simulink model "DFA_PID_Controller_ESC"  (R2014a)
settings: Solver=ode4  StartTime=0.0  StopTime=Tfinal  FixedStep=Tstep  MaxStep=Tstep  RelTol=1e-7
values from neighbouring files (symbols this model uses):
  Accelmean = 0    [Script_DFA_PID_Controller_ESC.m]
  alpha0 = 0    [Script_DFA_PID_Controller_ESC.m]
  alpha_desired = 0.1    [Script_DFA_PID_Controller_ESC.m]
  beta0 = 0    [Script_DFA_PID_Controller_ESC.m]
  ci = [-.01235; -.01235; .01235; .01235]    [Script_DFA_PID_Controller_ESC.m]
  f0 = mg    [Script_DFA_PID_Controller_ESC.m]
  g = 9.806    [Script_DFA_PID_Controller_ESC.m]
  gamma0 = 0    [Script_DFA_PID_Controller_ESC.m]
  Gyromean = 0    [Script_DFA_PID_Controller_ESC.m]
  IR_mean = 0    [Script_DFA_PID_Controller_ESC.m]
  Ix = .004738    (= 0.004738)    [Script_DFA_PID_Controller_ESC.m]
  Ixy = Ix-Iy    (= -0.006032)    [Script_DFA_PID_Controller_ESC.m]
  Iy = .01077    (= 0.01077)    [Script_DFA_PID_Controller_ESC.m]
  Iyz = Iy-Iz    (= -0.0041)    [Script_DFA_PID_Controller_ESC.m]
  Iz = .01487    (= 0.01487)    [Script_DFA_PID_Controller_ESC.m]
  Izx = Iz-Ix    (= 0.010132)    [Script_DFA_PID_Controller_ESC.m]
  Kd_alpha = 60    [Script_DFA_PID_Controller_ESC.m]
  Kd_beta = 30    [Script_DFA_PID_Controller_ESC.m]
  Kd_gamma = 30    [Script_DFA_PID_Controller_ESC.m]
  Kd_x = 0.008    [Script_DFA_PID_Controller_ESC.m]
  Kd_y = 0.002    [Script_DFA_PID_Controller_ESC.m]
  Kd_z = 100    [Script_DFA_PID_Controller_ESC.m]
  Ki_alpha = 0    [Script_DFA_PID_Controller_ESC.m]
  Ki_beta = 0    [Script_DFA_PID_Controller_ESC.m]
  Ki_gamma = 0    [Script_DFA_PID_Controller_ESC.m]
  Ki_x = 0    [Script_DFA_PID_Controller_ESC.m]
  Ki_y = 0    [Script_DFA_PID_Controller_ESC.m]
  Ki_z = 200    [Script_DFA_PID_Controller_ESC.m]
  Kp_alpha = 50    [Script_DFA_PID_Controller_ESC.m]
  Kp_beta = 8    [Script_DFA_PID_Controller_ESC.m]
  Kp_gamma = 15    [Script_DFA_PID_Controller_ESC.m]
  Kp_x = .1    (= 0.1)    [Script_DFA_PID_Controller_ESC.m]
  Kp_y = .15    (= 0.15)    [Script_DFA_PID_Controller_ESC.m]
  Kp_z = 200    [Script_DFA_PID_Controller_ESC.m]
  m_total = sum(m)    [Script_DFA_PID_Controller_ESC.m]
  p0 = omega(1)    [Script_DFA_PID_Controller_ESC.m]
  poly_order = 1    [Script_DFA_PID_Controller_ESC.m]
  q0 = omega(2)    [Script_DFA_PID_Controller_ESC.m]
  r0 = omega(3)    [Script_DFA_PID_Controller_ESC.m]
  salpha = (2*10^-4)*(pi/180)    (= 3.49065850399e-06)    [Script_DFA_PID_Controller_ESC.m]
  salphadot = (5.7*10^-4)*(pi/180)    (= 9.94837673637e-06)    [Script_DFA_PID_Controller_ESC.m]
  sbeta = (2*10^-4)*(pi/180)    (= 3.49065850399e-06)    [Script_DFA_PID_Controller_ESC.m]
  sbetadot = (5.4*10^-4)*(pi/180)    (= 9.42477796077e-06)    [Script_DFA_PID_Controller_ESC.m]
  SENS_NOISE01 = 1    [Script_DFA_PID_Controller_ESC.m]
  sgamma = (2*10^-4)*(pi/180)    (= 3.49065850399e-06)    [Script_DFA_PID_Controller_ESC.m]
  sgammadot = (5.4*10^-4)*(pi/180)    (= 9.42477796077e-06)    [Script_DFA_PID_Controller_ESC.m]
  sx = (3*10^-4)/1000    (= 3e-07)    [Script_DFA_PID_Controller_ESC.m]
  sxdot = (3*10^-2)*(pi/180)    (= 0.000523598775598)    [Script_DFA_PID_Controller_ESC.m]
  sy = (3*10^-4)/1000    (= 3e-07)    [Script_DFA_PID_Controller_ESC.m]
  sydot = (3*10^-2)*(pi/180)    (= 0.000523598775598)    [Script_DFA_PID_Controller_ESC.m]
  sz = (5.8*10^-3)/1000    (= 5.8e-06)    [Script_DFA_PID_Controller_ESC.m]
  ThreeD_mean = 0    [Script_DFA_PID_Controller_ESC.m]
  vect_xi = [ -.154;     .154;      0;      0]    [Script_DFA_PID_Controller_ESC.m]
  vect_yi = [     0;        0;   .087;  -.087]    [Script_DFA_PID_Controller_ESC.m]
  x0 = 0    [Script_DFA_PID_Controller_ESC.m]
  x0dot = 0    [Script_DFA_PID_Controller_ESC.m]
  y0 = 0    [Script_DFA_PID_Controller_ESC.m]
  y0dot = 0    [Script_DFA_PID_Controller_ESC.m]
  z0 = 0    [Script_DFA_PID_Controller_ESC.m]
  z0dot = 0    [Script_DFA_PID_Controller_ESC.m]
  z_desired = 0.25    [Script_DFA_PID_Controller_ESC.m]
settings Model: Creator=colempT430  LastModifiedBy=Young
settings DataIOCC: SignalLoggingSaveFormat=ModelDataLogs
settings OptimizationCC: ExpressionDepthLimit=2147483647
settings DebuggingCC: UnderspecifiedInitializationDetection=Classic  FcnCallInpInsideContextMsg=EnableAllAsWarning  StateNameClashWarn=warning

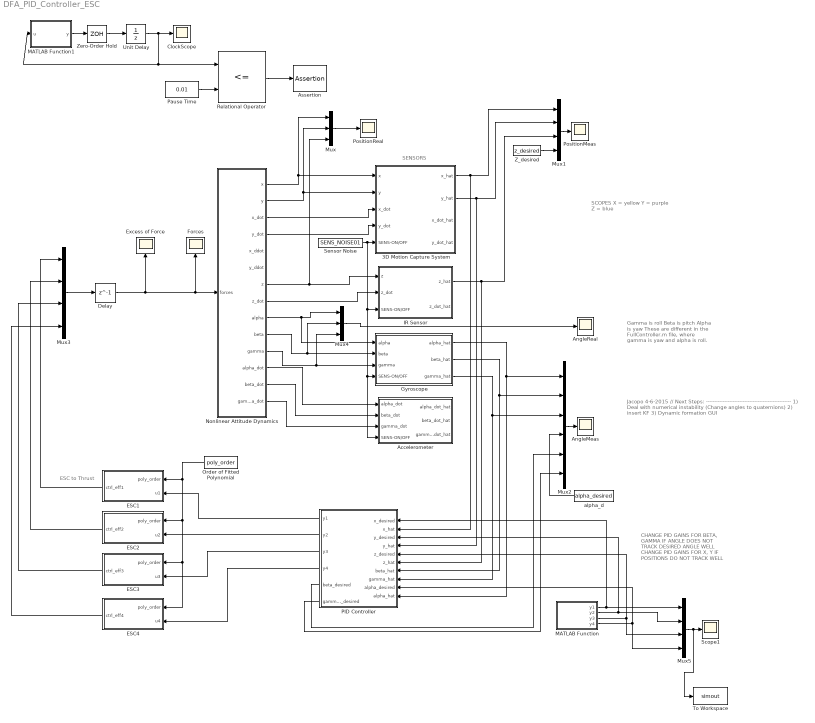
== system DFA_PID_Controller_ESC ==
  note: CHANGE PID GAINS FOR
      | BETA, GAMMA IF ANGLE
      | DOES NOT TRACK DESIRED
      | ANGLE WELL
      |
      | CHANGE PID GAINS FOR
      | X, Y IF POSITIONS DO NOT
      | TRACK WELL
  note: ESC to Thrust
  note: SENSORS
  note: SCOPES
      |
      | X = yellow
      | Y = purple
      | Z = blue
  note: Gamma is roll
      | Beta is pitch
      | Alpha is yaw
      |
      | These are different in the FullController.m file, where gamma is yaw and alpha is roll.
  note: Jacopo 4-6-2015 // Next Steps:
      | ---------------------------------------------------
      | 1) Deal with numerical instability (Change angles to quaternions)
      | 2) insert KF
      | 3) Dynamic formation GUI
  3D Motion Capture System : Subsystem
  Accelerometer : Subsystem
  AngleMeas : Scope
      settings: YMin=-0.25  YMax=0.4  SaveName=PositionMeas1
  AngleReal : Scope
      settings: YMin=-0.25  YMax=0.4  SaveName=PositionMeas2
  Assertion : Assertion  AssertionFailFcn=set_param(bdroot, 'SimulationCommand', 'pause')  StopWhenAssertionFail=off
  ClockScope : Scope
      settings: SaveName=NclockData
  Delay : Delay  DelayLength=1  InitialCondition=f0
  ESC1 : MATLAB Function  TreatAsAtomicUnit=on
  ESC2 : MATLAB Function  TreatAsAtomicUnit=on
  ESC3 : MATLAB Function  TreatAsAtomicUnit=on
  ESC4 : MATLAB Function  TreatAsAtomicUnit=on
  Excess of Force : Scope
      settings: SaveName=input_u
  Forces : Scope
      settings: SaveName=input_u1
  Gyroscope : Subsystem
  IR Sensor : Subsystem
  MATLAB Function : MATLAB Function  TreatAsAtomicUnit=on
  MATLAB Function1 : MATLAB Function  TreatAsAtomicUnit=on
  Mux : Mux  Inputs=3
  Mux1 : Mux
  Mux2 : Mux  Inputs=6
  Mux3 : Mux
  Mux4 : Mux  Inputs=3
  Mux5 : Mux
  Nonlinear Attitude Dynamics : Subsystem
  Order of Fitted Polynomial : Constant  Value=poly_order
  PID Controller : Subsystem
  Pause Time : Constant  Value=0.01
  PositionMeas : Scope
      settings: YMin=-0.025  YMax=0.5  SaveName=PositionMeas
  PositionReal : Scope
      settings: YMin=0  YMax=0.275  SaveName=PositionReal
  Relational Operator : RelationalOperator  Operator=<=  OutDataTypeStr=boolean
  Scope1 : Scope
  Sensor Noise : Constant  Value=SENS_NOISE01
  To Workspace : ToWorkspace  VariableName=simout  SampleTime=-1
      settings: Save2DSignal=2-D array (concatenate along first dimension)
  Unit Delay : UnitDelay  SampleTime=-1
  Z_desired : Constant  Value=z_desired
  Zero-Order Hold : ZeroOrderHold  SampleTime=-1
  alpha_d : Constant  Value=alpha_desired
  wires:
  Nonlinear Attitude Dynamics/1(x) -> 3D Motion Capture System/1(x), Mux/1
  Nonlinear Attitude Dynamics/2(y) -> 3D Motion Capture System/2(y), Mux/2
  Nonlinear Attitude Dynamics/7(z) -> IR Sensor/1(z), Mux/3
  Nonlinear Attitude Dynamics/9(alpha) -> Gyroscope/1(alpha), Mux4/1
  Nonlinear Attitude Dynamics/10(beta) -> Gyroscope/2(beta), Mux4/2
  Nonlinear Attitude Dynamics/11(gamma) -> Gyroscope/3(gamma), Mux4/3
  Nonlinear Attitude Dynamics/13(beta_dot) -> Accelerometer/2(beta_dot)
  3D Motion Capture System/1(x_hat) -> PID Controller/2(x_hat), Mux1/1
  IR Sensor/1(z_hat) -> PID Controller/6(z_hat), Mux1/3
  3D Motion Capture System/2(y_hat) -> PID Controller/4(y_hat), Mux1/2
  Gyroscope/2(beta_hat) -> PID Controller/7(beta_hat), Mux2/2
  Nonlinear Attitude Dynamics/3(x_dot) -> 3D Motion Capture System/3(x_dot)
  Nonlinear Attitude Dynamics/4(y_dot) -> 3D Motion Capture System/4(y_dot)
  Nonlinear Attitude Dynamics/8(z_dot) -> IR Sensor/2(z_dot)
  Mux/1 -> PositionReal/1
  Mux1/1 -> PositionMeas/1
  Sensor Noise/1 -> 3D Motion Capture System/5(SENS-ON/OFF), Accelerometer/4(SENS-ON/OFF), Gyroscope/4(SENS-ON/OFF), IR Sensor/3(SENS-ON/OFF)
  Gyroscope/1(alpha_hat) -> PID Controller/10(alpha_hat), Mux2/1
  Gyroscope/3(gamma_hat) -> Mux2/3, PID Controller/8(gamma_hat)
  MATLAB Function/4(y4) -> Mux5/4, PID Controller/9(alpha_desired)
  Mux2/1 -> AngleMeas/1
  Z_desired/1 -> Mux1/4
  alpha_d/1 -> Mux2/4
  PID Controller/5(beta_desired) -> Mux2/5
  PID Controller/6(gamma_desired) -> Mux2/6
  Nonlinear Attitude Dynamics/12(alpha_dot) -> Accelerometer/1(alpha_dot)
  Nonlinear Attitude Dynamics/14(gamma_dot) -> Accelerometer/3(gamma_dot)
  MATLAB Function/1(y1) -> Mux5/1, PID Controller/1(x_desired)
  Order of Fitted Polynomial/1 -> ESC4/1(poly_order), ESC3/1(poly_order), ESC2/1(poly_order), ESC1/1(poly_order)
  Delay/1 -> Forces/1, Nonlinear Attitude Dynamics/1(forces), Excess of Force/1
  Mux3/1 -> Delay/1
  ESC2/1(ctrl_eff2) -> Mux3/2
  ESC3/1(ctrl_eff3) -> Mux3/3
  ESC4/1(ctrl_eff4) -> Mux3/4
  ESC1/1(ctrl_eff1) -> Mux3/1
  PID Controller/1(y1) -> ESC1/2(u1)
  PID Controller/2(y2) -> ESC2/2(u2)
  PID Controller/3(y3) -> ESC3/2(u3)
  PID Controller/4(y4) -> ESC4/2(u4)
  Mux4/1 -> AngleReal/1
  MATLAB Function/2(y2) -> Mux5/2, PID Controller/3(y_desired)
  MATLAB Function/3(y3) -> Mux5/3, PID Controller/5(z_desired)
  Pause Time/1 -> Relational Operator/2
  Relational Operator/1 -> Assertion/1
  Zero-Order Hold/1 -> Unit Delay/1
  MATLAB Function1/1(y) -> Zero-Order Hold/1
  Unit Delay/1 -> Relational Operator/1, MATLAB Function1/1(u), ClockScope/1
  Mux5/1 -> To Workspace/1, Scope1/1

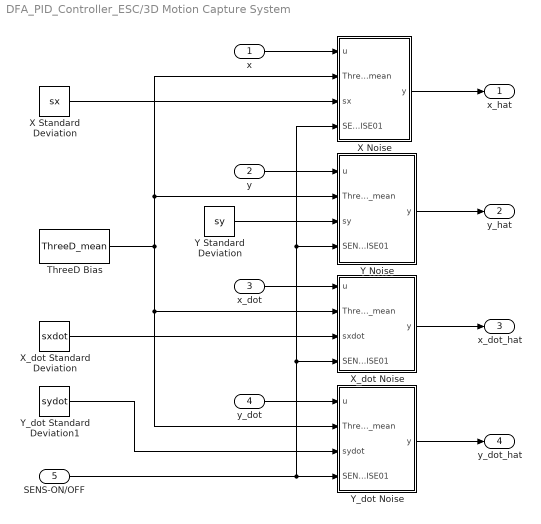
== system DFA_PID_Controller_ESC/3D Motion Capture System ==
  x : Inport
  y : Inport  Port=2
  x_dot : Inport  Port=3
  y_dot : Inport  Port=4
  SENS-ON/OFF : Inport  Port=5
  ThreeD Bias : Constant  Value=ThreeD_mean
  X Noise : MATLAB Function  TreatAsAtomicUnit=on
  X Standard Deviation : Constant  Value=sx
  X_dot Noise : MATLAB Function  TreatAsAtomicUnit=on
  X_dot Standard Deviation : Constant  Value=sxdot
  Y Noise : MATLAB Function  TreatAsAtomicUnit=on
  Y Standard Deviation : Constant  Value=sy
  Y_dot Noise : MATLAB Function  TreatAsAtomicUnit=on
  Y_dot Standard Deviation1 : Constant  Value=sydot
  x_hat : Outport
  y_hat : Outport  Port=2
  x_dot_hat : Outport  Port=3
  y_dot_hat : Outport  Port=4
  wires:
  x/1 -> X Noise/1(u)
  X Noise/1(y) -> x_hat/1
  y/1 -> Y Noise/1(u)
  Y Noise/1(y) -> y_hat/1
  x_dot/1 -> X_dot Noise/1(u)
  X_dot Noise/1(y) -> x_dot_hat/1
  y_dot/1 -> Y_dot Noise/1(u)
  Y_dot Noise/1(y) -> y_dot_hat/1
  X Standard Deviation/1 -> X Noise/3(sx)
  X_dot Standard Deviation/1 -> X_dot Noise/3(sxdot)
  ThreeD Bias/1 -> X Noise/2(ThreeD_mean), Y Noise/2(ThreeD_mean), Y_dot Noise/2(ThreeD_mean), X_dot Noise/2(ThreeD_mean)
  SENS-ON/OFF/1 -> X Noise/4(SENS_NOISE01), Y Noise/4(SENS_NOISE01), X_dot Noise/4(SENS_NOISE01), Y_dot Noise/4(SENS_NOISE01)
  Y Standard Deviation/1 -> Y Noise/3(sy)
  Y_dot Standard Deviation1/1 -> Y_dot Noise/3(sydot)

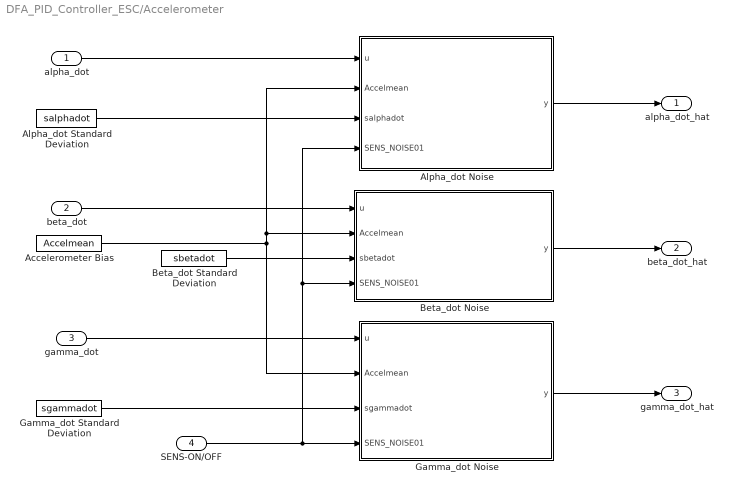
== system DFA_PID_Controller_ESC/Accelerometer ==
  alpha_dot : Inport
  beta_dot : Inport  Port=2
  gamma_dot : Inport  Port=3
  SENS-ON/OFF : Inport  Port=4
  Accelerometer Bias : Constant  Value=Accelmean
  Alpha_dot Noise : MATLAB Function  TreatAsAtomicUnit=on
  Alpha_dot Standard Deviation : Constant  Value=salphadot
  Beta_dot Noise : MATLAB Function  TreatAsAtomicUnit=on
  Beta_dot Standard Deviation : Constant  Value=sbetadot
  Gamma_dot Noise : MATLAB Function  TreatAsAtomicUnit=on
  Gamma_dot Standard Deviation : Constant  Value=sgammadot
  alpha_dot_hat : Outport
  beta_dot_hat : Outport  Port=2
  gamma_dot_hat : Outport  Port=3
  wires:
  beta_dot/1 -> Beta_dot Noise/1(u)
  gamma_dot/1 -> Gamma_dot Noise/1(u)
  Beta_dot Noise/1(y) -> beta_dot_hat/1
  Gamma_dot Noise/1(y) -> gamma_dot_hat/1
  alpha_dot/1 -> Alpha_dot Noise/1(u)
  Alpha_dot Noise/1(y) -> alpha_dot_hat/1
  Accelerometer Bias/1 -> Alpha_dot Noise/2(Accelmean), Beta_dot Noise/2(Accelmean), Gamma_dot Noise/2(Accelmean)
  Gamma_dot Standard Deviation/1 -> Gamma_dot Noise/3(sgammadot)
  Alpha_dot Standard Deviation/1 -> Alpha_dot Noise/3(salphadot)
  Beta_dot Standard Deviation/1 -> Beta_dot Noise/3(sbetadot)
  SENS-ON/OFF/1 -> Gamma_dot Noise/4(SENS_NOISE01), Beta_dot Noise/4(SENS_NOISE01), Alpha_dot Noise/4(SENS_NOISE01)

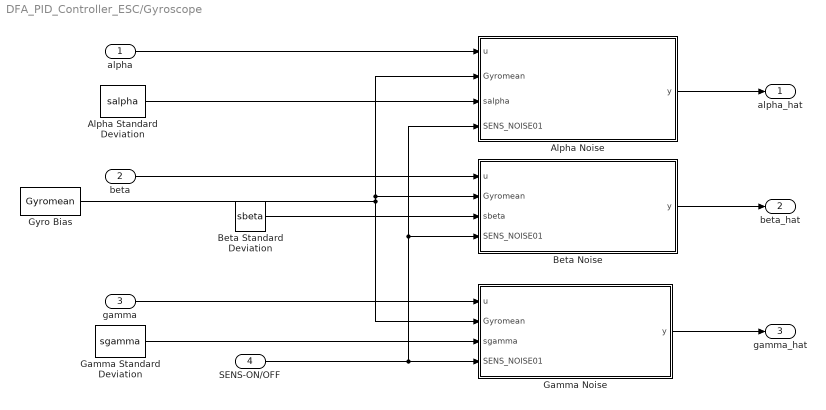
== system DFA_PID_Controller_ESC/Gyroscope ==
  alpha : Inport
  beta : Inport  Port=2
  gamma : Inport  Port=3
  SENS-ON/OFF : Inport  Port=4
  Alpha Noise : MATLAB Function  TreatAsAtomicUnit=on
  Alpha Standard Deviation : Constant  Value=salpha
  Beta Noise : MATLAB Function  TreatAsAtomicUnit=on
  Beta Standard Deviation : Constant  Value=sbeta
  Gamma Noise : MATLAB Function  TreatAsAtomicUnit=on
  Gamma Standard Deviation : Constant  Value=sgamma
  Gyro Bias : Constant  Value=Gyromean
  alpha_hat : Outport
  beta_hat : Outport  Port=2
  gamma_hat : Outport  Port=3
  wires:
  gamma/1 -> Gamma Noise/1(u)
  Gamma Noise/1(y) -> gamma_hat/1
  Alpha Noise/1(y) -> alpha_hat/1
  Beta Noise/1(y) -> beta_hat/1
  beta/1 -> Beta Noise/1(u)
  alpha/1 -> Alpha Noise/1(u)
  Alpha Standard Deviation/1 -> Alpha Noise/3(salpha)
  Beta Standard Deviation/1 -> Beta Noise/3(sbeta)
  Gamma Standard Deviation/1 -> Gamma Noise/3(sgamma)
  Gyro Bias/1 -> Alpha Noise/2(Gyromean), Beta Noise/2(Gyromean), Gamma Noise/2(Gyromean)
  SENS-ON/OFF/1 -> Beta Noise/4(SENS_NOISE01), Alpha Noise/4(SENS_NOISE01), Gamma Noise/4(SENS_NOISE01)

== system DFA_PID_Controller_ESC/IR Sensor ==
  z : Inport
  z_dot : Inport  Port=2
  SENS-ON/OFF : Inport  Port=3
  IR Bias : Constant  Value=IR_mean
  Z Noise : MATLAB Function  TreatAsAtomicUnit=on
  Z Standard Deviation : Constant  Value=sz
  Z_dot Noise : MATLAB Function  TreatAsAtomicUnit=on
  z_hat : Outport
  z_dot_hat : Outport  Port=2
  wires:
  z/1 -> Z Noise/1(u)
  Z Noise/1(y) -> z_hat/1
  z_dot/1 -> Z_dot Noise/1(u)
  Z_dot Noise/1(y) -> z_dot_hat/1
  Z Standard Deviation/1 -> Z_dot Noise/3(sz), Z Noise/3(sz)
  IR Bias/1 -> Z_dot Noise/2(IR_mean), Z Noise/2(IR_mean)
  SENS-ON/OFF/1 -> Z_dot Noise/4(SENS_NOISE01), Z Noise/4(SENS_NOISE01)

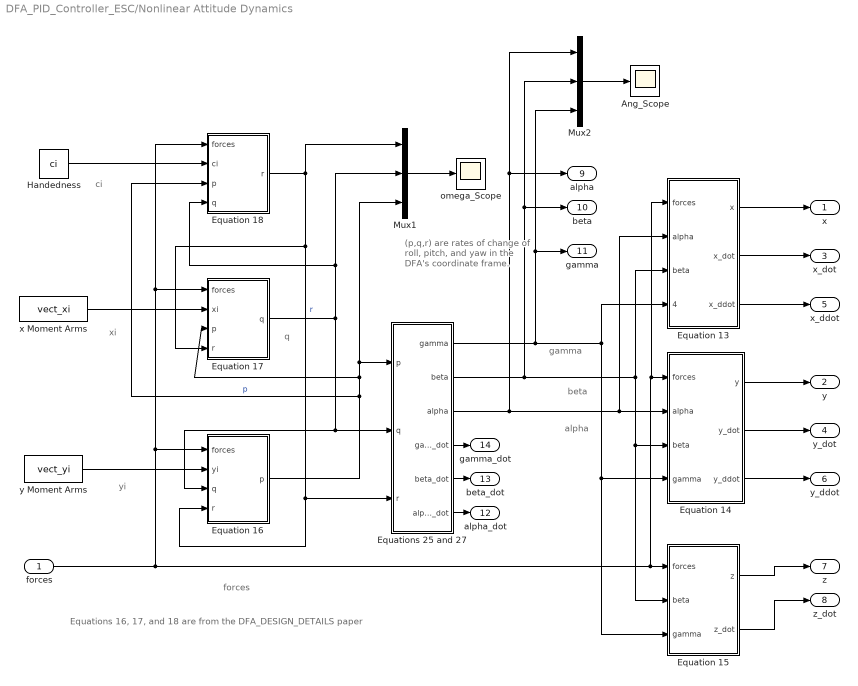
== system DFA_PID_Controller_ESC/Nonlinear Attitude Dynamics ==
  note: gamma
  note: Equations 16, 17, and 18 are from the DFA_DESIGN_DETAILS paper
  note: (p,q,r) are rates of change of roll, pitch, and yaw in the DFA's coordinate frame.
  note: forces
  note: yi
  note: xi
  note: ci
  note: q
  note: beta
  note: alpha
  forces : Inport
  Ang_Scope : Scope
      settings: SaveName=Ang_Scope1
  Equation 13 : Subsystem
  Equation 14 : Subsystem
  Equation 15 : Subsystem
  Equation 16 : Subsystem
  Equation 17 : Subsystem
  Equation 18 : Subsystem
  Equations 25 and 27 : Subsystem
  Handedness : Constant  Value=ci
  Mux1 : Mux  Inputs=3
  Mux2 : Mux  Inputs=3
  omega_Scope : Scope
      settings: SaveName=angle_Scope1
  x Moment Arms : Constant  Value=vect_xi
  y Moment Arms : Constant  Value=vect_yi
  x : Outport
  y : Outport  Port=2
  x_dot : Outport  Port=3
  y_dot : Outport  Port=4
  x_ddot : Outport  Port=5
  y_ddot : Outport  Port=6
  z : Outport  Port=7
  z_dot : Outport  Port=8
  alpha : Outport  Port=9
  beta : Outport  Port=10
  gamma : Outport  Port=11
  alpha_dot : Outport  Port=12
  beta_dot : Outport  Port=13
  gamma_dot : Outport  Port=14
  wires:
  Equation 18/1(r) -> Equations 25 and 27/3(r), Equation 16/4(r), Equation 17/4(r), Mux1/1  "r"
  Equation 16/1(p) -> Equation 18/3(p), Equations 25 and 27/1(p), Mux1/3, Equation 17/3(p)  "p"
  Handedness/1 -> Equation 18/2(ci)
  Equation 13/1(x) -> x/1
  Equation 14/1(y) -> y/1
  Equation 15/1(z) -> z/1
  Mux1/1 -> omega_Scope/1
  x Moment Arms/1 -> Equation 17/2(xi)
  Equation 17/1(q) -> Equations 25 and 27/2(q), Equation 16/3(q), Equation 18/4(q), Mux1/2
  y Moment Arms/1 -> Equation 16/2(yi)
  Equations 25 and 27/1(gamma) -> Equation 15/3(gamma), Equation 14/4(gamma), Equation 13/4(gamma), Mux2/3, gamma/1
  Equations 25 and 27/2(beta) -> Equation 15/2(beta), Equation 14/3(beta), Equation 13/3(beta), Mux2/2, beta/1
  Equations 25 and 27/3(alpha) -> Equation 13/2(alpha), Equation 14/2(alpha), Mux2/1, alpha/1
  Equations 25 and 27/4(gamma_dot) -> gamma_dot/1
  Equations 25 and 27/5(beta_dot) -> beta_dot/1
  Equations 25 and 27/6(alpha_dot) -> alpha_dot/1
  Equation 13/2(x_dot) -> x_dot/1
  Equation 14/2(y_dot) -> y_dot/1
  Equation 15/2(z_dot) -> z_dot/1
  forces/1 -> Equation 18/1(forces), Equation 17/1(forces), Equation 16/1(forces), Equation 13/1(forces), Equation 14/1(forces), Equation 15/1(forces)
  Mux2/1 -> Ang_Scope/1
  Equation 13/3(x_ddot) -> x_ddot/1
  Equation 14/3(y_ddot) -> y_ddot/1

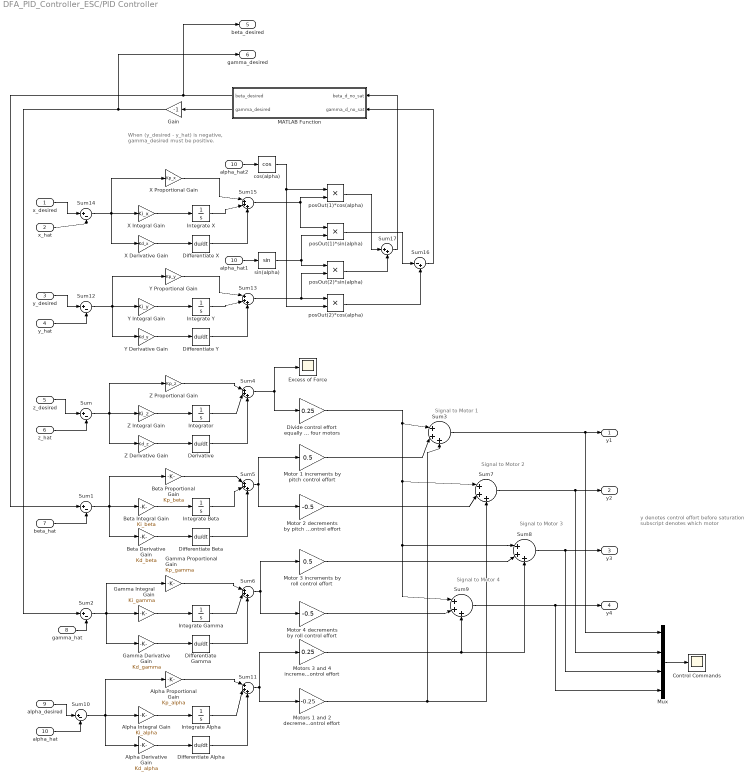
== system DFA_PID_Controller_ESC/PID Controller ==
  note: When (y_desired - y_hat) is negative,
      | gamma_desired must be positive.
  note: y denotes control effort before saturation
      | subscript denotes which motor
  note: Signal to Motor 4
  note: Signal to Motor 3
  note: Signal to Motor 2
  note: Signal to Motor 1
  x_desired : Inport
  x_hat : Inport  Port=2
  y_desired : Inport  Port=3
  y_hat : Inport  Port=4
  z_desired : Inport  Port=5
  z_hat : Inport  Port=6
  beta_hat : Inport  Port=7
  gamma_hat : Inport  Port=8
  alpha_desired : Inport  Port=9
  alpha_hat : Inport  Port=10
  Alpha Derivative Gain : Gain  Gain=Kd_alpha
  Alpha Integral Gain : Gain  Gain=Ki_alpha
  Alpha Proportional Gain : Gain  Gain=Kp_alpha
  Beta Derivative Gain : Gain  Gain=Kd_beta
  Beta Integral Gain : Gain  Gain=Ki_beta
  Beta Proportional Gain : Gain  Gain=Kp_beta
  Control Commands : Scope
      settings: SaveName=ControlCommandScope
  Derivative : Derivative
  Differentiate Alpha : Derivative
  Differentiate Beta : Derivative
  Differentiate Gamma : Derivative
  Differentiate X : Derivative
  Differentiate Y : Derivative
  Divide control effort equally among the four motors : Gain  Gain=0.25
  Excess of Force : Scope
      settings: SaveName=ExcessForce
  Gain : Gain  Gain=-1
  Gamma Derivative Gain : Gain  Gain=Kd_gamma
  Gamma Integral Gain : Gain  Gain=Ki_gamma
  Gamma Proportional Gain : Gain  Gain=Kp_gamma
  Integrate Alpha : Integrator
  Integrate Beta : Integrator
  Integrate Gamma : Integrator
  Integrate X : Integrator
  Integrate Y : Integrator
  Integrator : Integrator
  MATLAB Function : MATLAB Function  TreatAsAtomicUnit=on
  Motor 1 increments by pitch control effort : Gain  Gain=0.5
  Motor 2 decrements by pitch control effort : Gain  Gain=-0.5
  Motor 3 increments by roll control effort : Gain  Gain=0.5
  Motor 4 decrements by roll control effort : Gain  Gain=-0.5
  Motors 1 and 2 decrement by the pitch control effort : Gain  Gain=-0.25
  Motors 3 and 4 increment by the pitch control effort : Gain  Gain=0.25
  Mux : Mux
  Sum{,1..2,10,12,14} (6 alike) : Sum  Inputs=|+-
  Sum{3..9,11,13,15} (10 alike) : Sum  Inputs=|+++
  Sum16 : Sum  Inputs=|-+
  Sum17 : Sum  Inputs=|++
  X Derivative Gain : Gain  Gain=Kd_x
  X Integral Gain : Gain  Gain=Ki_x
  X Proportional Gain : Gain  Gain=Kp_x
  Y Derivative Gain : Gain  Gain=Kd_y
  Y Integral Gain : Gain  Gain=Ki_y
  Y Proportional Gain : Gain  Gain=Kp_y
  Z Derivative Gain : Gain  Gain=Kd_z
  Z Integral Gain : Gain  Gain=Ki_z
  Z Proportional Gain : Gain  Gain=Kp_z
  alpha_hat1 : InportShadow  Port=10
  alpha_hat2 : InportShadow  Port=10
  cos(alpha) : Trigonometry  Operator=cos
  posOut(1)*cos(alpha) : Product
  posOut(1)*sin(alpha) : Product
  posOut(2)*cos(alpha) : Product
  posOut(2)*sin(alpha) : Product
  sin(alpha) : Trigonometry
  y1 : Outport
  y2 : Outport  Port=2
  y3 : Outport  Port=3
  y4 : Outport  Port=4
  beta_desired : Outport  Port=5
  gamma_desired : Outport  Port=6
  wires:
  z_desired/1 -> Sum/1
  z_hat/1 -> Sum/2
  beta_hat/1 -> Sum1/2
  gamma_hat/1 -> Sum2/2
  Sum/1 -> Z Derivative Gain/1, Z Integral Gain/1, Z Proportional Gain/1
  Sum1/1 -> Beta Derivative Gain/1, Beta Proportional Gain/1, Beta Integral Gain/1
  Sum2/1 -> Gamma Derivative Gain/1, Gamma Proportional Gain/1, Gamma Integral Gain/1
  Z Integral Gain/1 -> Integrator/1
  Z Proportional Gain/1 -> Sum4/1
  Integrator/1 -> Sum4/2
  Beta Proportional Gain/1 -> Sum5/1
  Beta Integral Gain/1 -> Integrate Beta/1
  Integrate Beta/1 -> Sum5/2
  Gamma Integral Gain/1 -> Integrate Gamma/1
  Gamma Proportional Gain/1 -> Sum6/1
  Integrate Gamma/1 -> Sum6/2
  Sum5/1 -> Motor 2 decrements by pitch control effort/1, Motor 1 increments by pitch control effort/1
  Divide control effort equally among the four motors/1 -> Sum8/1, Sum9/1, Sum7/1, Sum3/1
  Sum3/1 -> y1/1, Mux/1
  Sum7/1 -> y2/1, Mux/2
  Sum8/1 -> y3/1, Mux/3
  Sum9/1 -> y4/1, Mux/4
  Mux/1 -> Control Commands/1
  Z Derivative Gain/1 -> Derivative/1
  Derivative/1 -> Sum4/3
  Gamma Derivative Gain/1 -> Differentiate Gamma/1
  Sum6/1 -> Motor 4 decrements by roll control effort/1, Motor 3 increments by roll control effort/1
  Differentiate Gamma/1 -> Sum6/3
  Beta Derivative Gain/1 -> Differentiate Beta/1
  Differentiate Beta/1 -> Sum5/3
  alpha_desired/1 -> Sum10/1
  alpha_hat/1 -> Sum10/2
  Sum10/1 -> Alpha Derivative Gain/1, Alpha Proportional Gain/1, Alpha Integral Gain/1
  Alpha Integral Gain/1 -> Integrate Alpha/1
  Integrate Alpha/1 -> Sum11/2
  Alpha Proportional Gain/1 -> Sum11/1
  Alpha Derivative Gain/1 -> Differentiate Alpha/1
  Differentiate Alpha/1 -> Sum11/3
  y_desired/1 -> Sum12/1
  y_hat/1 -> Sum12/2
  Sum12/1 -> Y Derivative Gain/1, Y Proportional Gain/1, Y Integral Gain/1
  Y Integral Gain/1 -> Integrate Y/1
  Integrate Y/1 -> Sum13/2
  Y Proportional Gain/1 -> Sum13/1
  Y Derivative Gain/1 -> Differentiate Y/1
  Differentiate Y/1 -> Sum13/3
  x_desired/1 -> Sum14/1
  x_hat/1 -> Sum14/2
  Sum14/1 -> X Derivative Gain/1, X Proportional Gain/1, X Integral Gain/1
  X Integral Gain/1 -> Integrate X/1
  Integrate X/1 -> Sum15/2
  X Proportional Gain/1 -> Sum15/1
  X Derivative Gain/1 -> Differentiate X/1
  Differentiate X/1 -> Sum15/3
  Sum11/1 -> Motors 1 and 2 decrement by the pitch control effort/1, Motors 3 and 4 increment by the pitch control effort/1
  Motors 3 and 4 increment by the pitch control effort/1 -> Sum8/3, Sum9/3
  Motors 1 and 2 decrement by the pitch control effort/1 -> Sum7/3, Sum3/3
  Motor 1 increments by pitch control effort/1 -> Sum3/2
  Motor 2 decrements by pitch control effort/1 -> Sum7/2
  Motor 3 increments by roll control effort/1 -> Sum8/2
  Motor 4 decrements by roll control effort/1 -> Sum9/2
  alpha_hat1/1 -> sin(alpha)/1
  Sum15/1 -> posOut(1)*cos(alpha)/2, posOut(1)*sin(alpha)/1
  sin(alpha)/1 -> posOut(2)*sin(alpha)/1, posOut(1)*sin(alpha)/2
  Sum13/1 -> posOut(2)*cos(alpha)/1, posOut(2)*sin(alpha)/2
  alpha_hat2/1 -> cos(alpha)/1
  cos(alpha)/1 -> posOut(2)*cos(alpha)/2, posOut(1)*cos(alpha)/1
  posOut(2)*cos(alpha)/1 -> Sum16/2
  posOut(1)*sin(alpha)/1 -> Sum16/1
  posOut(1)*cos(alpha)/1 -> Sum17/1
  posOut(2)*sin(alpha)/1 -> Sum17/2
  Sum4/1 -> Divide control effort equally among the four motors/1, Excess of Force/1
  Sum17/1 -> MATLAB Function/1(beta_d_no_sat)
  Sum16/1 -> MATLAB Function/2(gamma_d_no_sat)
  MATLAB Function/2(gamma_desired) -> Gain/1
  MATLAB Function/1(beta_desired) -> beta_desired/1, Sum1/1
  Gain/1 -> Sum2/1, gamma_desired/1

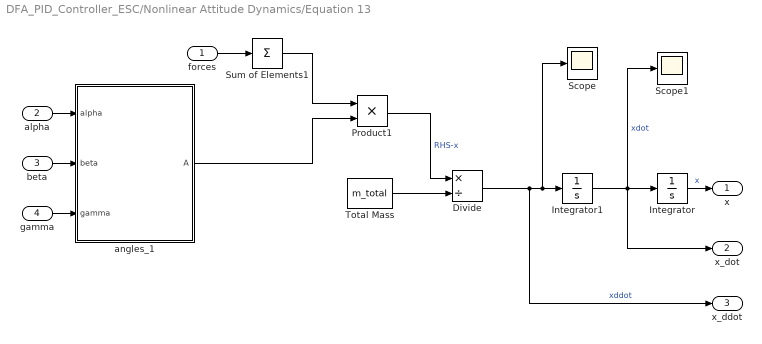
== system DFA_PID_Controller_ESC/Nonlinear Attitude Dynamics/Equation 13 ==
  forces : Inport
  alpha : Inport  Port=2
  beta : Inport  Port=3
  gamma : Inport  Port=4
  Divide : Product  Inputs=*/
  Integrator : Integrator  InitialCondition=x0
  Integrator1 : Integrator  InitialCondition=x0dot
  Product1 : Product  RndMeth=Zero
  Scope : Scope
      settings: SaveName=xddot
  Scope1 : Scope
      settings: SaveName=xdot
  Sum of Elements1 : Sum  Inputs=+
  Total Mass : Constant  Value=m_total
  angles_1 : MATLAB Function  TreatAsAtomicUnit=on
  x : Outport
  x_dot : Outport  Port=2
  x_ddot : Outport  Port=3
  wires:
  Sum of Elements1/1 -> Product1/1
  forces/1 -> Sum of Elements1/1
  Product1/1 -> Divide/1  "RHS-x"
  gamma/1 -> angles_1/3(gamma)
  Integrator/1 -> x/1  "x"
  beta/1 -> angles_1/2(beta)
  alpha/1 -> angles_1/1(alpha)
  Integrator1/1 -> Scope1/1, Integrator/1, x_dot/1  "xdot"
  Divide/1 -> x_ddot/1, Scope/1, Integrator1/1  "xddot"
  Total Mass/1 -> Divide/2
  angles_1/1(A) -> Product1/2

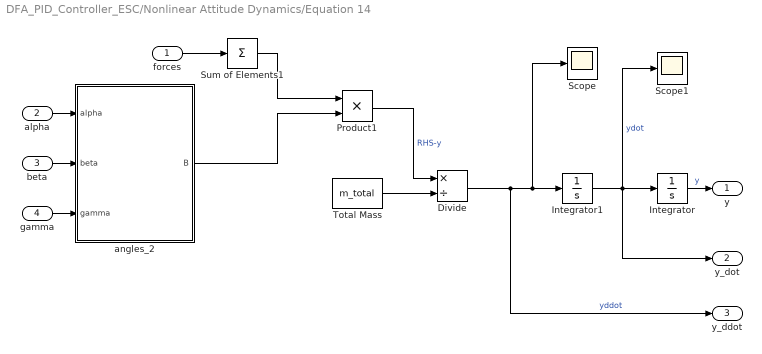
== system DFA_PID_Controller_ESC/Nonlinear Attitude Dynamics/Equation 14 ==
  forces : Inport
  alpha : Inport  Port=2
  beta : Inport  Port=3
  gamma : Inport  Port=4
  Divide : Product  Inputs=*/
  Integrator : Integrator  InitialCondition=y0
  Integrator1 : Integrator  InitialCondition=y0dot
  Product1 : Product  RndMeth=Zero
  Scope : Scope
      settings: SaveName=yddot
  Scope1 : Scope
      settings: SaveName=ydot
  Sum of Elements1 : Sum  Inputs=+
  Total Mass : Constant  Value=m_total
  angles_2 : MATLAB Function  TreatAsAtomicUnit=on
  y : Outport
  y_dot : Outport  Port=2
  y_ddot : Outport  Port=3
  wires:
  Sum of Elements1/1 -> Product1/1
  forces/1 -> Sum of Elements1/1
  Product1/1 -> Divide/1  "RHS-y"
  angles_2/1(B) -> Product1/2
  Total Mass/1 -> Divide/2
  Divide/1 -> y_ddot/1, Scope/1, Integrator1/1  "yddot"
  Integrator1/1 -> Scope1/1, Integrator/1, y_dot/1  "ydot"
  alpha/1 -> angles_2/1(alpha)
  beta/1 -> angles_2/2(beta)
  Integrator/1 -> y/1  "y"
  gamma/1 -> angles_2/3(gamma)

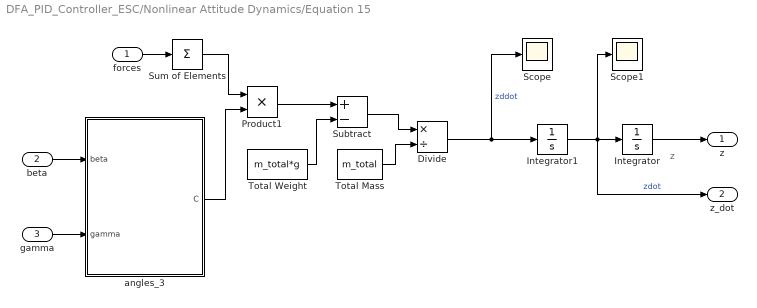
== system DFA_PID_Controller_ESC/Nonlinear Attitude Dynamics/Equation 15 ==
  note: z
  forces : Inport
  beta : Inport  Port=2
  gamma : Inport  Port=3
  Divide : Product  Inputs=*/
  Integrator : Integrator  InitialCondition=z0
  Integrator1 : Integrator  InitialCondition=z0dot
  Product1 : Product  RndMeth=Zero
  Scope : Scope
      settings: SaveName=zddot
  Scope1 : Scope
      settings: SaveName=zdot
  Subtract : Sum  Inputs=+-
  Sum of Elements : Sum  Inputs=+
  Total Mass : Constant  Value=m_total
  Total Weight : Constant  Value=m_total*g
  angles_3 : MATLAB Function  TreatAsAtomicUnit=on
  z : Outport
  z_dot : Outport  Port=2
  wires:
  gamma/1 -> angles_3/2(gamma)
  beta/1 -> angles_3/1(beta)
  angles_3/1(C) -> Product1/2
  forces/1 -> Sum of Elements/1
  Integrator/1 -> z/1
  Integrator1/1 -> Scope1/1, Integrator/1, z_dot/1  "zdot"
  Divide/1 -> Integrator1/1, Scope/1  "zddot"
  Total Mass/1 -> Divide/2
  Sum of Elements/1 -> Product1/1
  Subtract/1 -> Divide/1
  Product1/1 -> Subtract/1
  Total Weight/1 -> Subtract/2

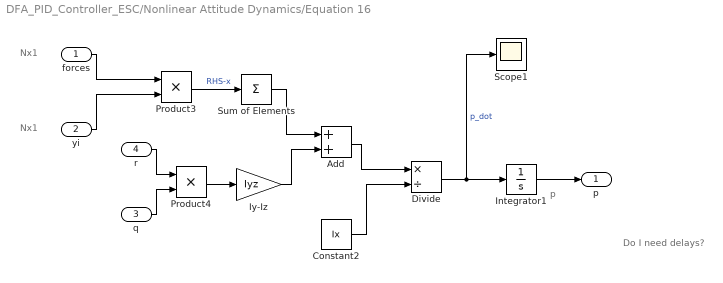
== system DFA_PID_Controller_ESC/Nonlinear Attitude Dynamics/Equation 16 ==
  note: Do I need delays?
  note: Nx1
  note: Nx1
  note: p
  forces : Inport
  yi : Inport  Port=2
  q : Inport  Port=3
  r : Inport  Port=4
  Add : Sum
  Constant2 : Constant  Value=Ix
  Divide : Product  Inputs=*/
  Integrator1 : Integrator  InitialCondition=p0
  Iy-Iz : Gain  Gain=Iyz
  Product3 : Product  RndMeth=Zero
  Product4 : Product  RndMeth=Zero
  Scope1 : Scope
      settings: SaveName=alphaddot3
  Sum of Elements : Sum  Inputs=+
  p : Outport
  wires:
  forces/1 -> Product3/1
  Integrator1/1 -> p/1
  Divide/1 -> Integrator1/1, Scope1/1  "p_dot"
  Constant2/1 -> Divide/2
  yi/1 -> Product3/2
  Product3/1 -> Sum of Elements/1  "RHS-x"
  r/1 -> Product4/1
  q/1 -> Product4/2
  Product4/1 -> Iy-Iz/1
  Sum of Elements/1 -> Add/1
  Iy-Iz/1 -> Add/2
  Add/1 -> Divide/1

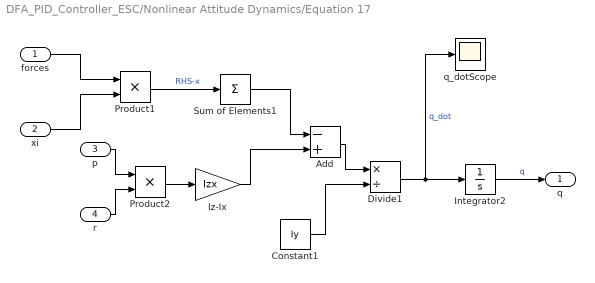
== system DFA_PID_Controller_ESC/Nonlinear Attitude Dynamics/Equation 17 ==
  forces : Inport
  xi : Inport  Port=2
  p : Inport  Port=3
  r : Inport  Port=4
  Add : Sum  Inputs=-+
  Constant1 : Constant  Value=Iy
  Divide1 : Product  Inputs=*/
  Integrator2 : Integrator  InitialCondition=q0
  Iz-Ix : Gain  Gain=Izx
  Product1 : Product  RndMeth=Zero
  Product2 : Product  RndMeth=Zero
  Sum of Elements1 : Sum  Inputs=+
  q_dotScope : Scope
      settings: SaveName=alphaddot1
  q : Outport
  wires:
  Sum of Elements1/1 -> Add/1
  Add/1 -> Divide1/1
  Iz-Ix/1 -> Add/2
  Product2/1 -> Iz-Ix/1
  r/1 -> Product2/2
  p/1 -> Product2/1
  Product1/1 -> Sum of Elements1/1  "RHS-x"
  xi/1 -> Product1/2
  Constant1/1 -> Divide1/2
  Divide1/1 -> q_dotScope/1, Integrator2/1  "q_dot"
  Integrator2/1 -> q/1  "q"
  forces/1 -> Product1/1

== system DFA_PID_Controller_ESC/Nonlinear Attitude Dynamics/Equation 18 ==
  forces : Inport
  ci : Inport  Port=2
  p : Inport  Port=3
  q : Inport  Port=4
  Add : Sum
  Constant : Constant  Value=Iz
  Divide : Product  Inputs=*/
  Integrator1 : Integrator  InitialCondition=r0
  Ix-Iy : Gain  Gain=Ixy
  Product : Product  RndMeth=Zero
  Product1 : Product  RndMeth=Zero
  Scope : Scope
      settings: SaveName=alphaddot
  Sum of Elements : Sum  Inputs=+
  r : Outport
  wires:
  Add/1 -> Divide/1
  Ix-Iy/1 -> Add/2
  Sum of Elements/1 -> Add/1
  Product1/1 -> Ix-Iy/1
  q/1 -> Product1/2
  p/1 -> Product1/1
  Product/1 -> Sum of Elements/1  "RHS-x"
  ci/1 -> Product/2
  Constant/1 -> Divide/2
  Divide/1 -> Integrator1/1, Scope/1  "r_dot"
  Integrator1/1 -> r/1  "r"
  forces/1 -> Product/1

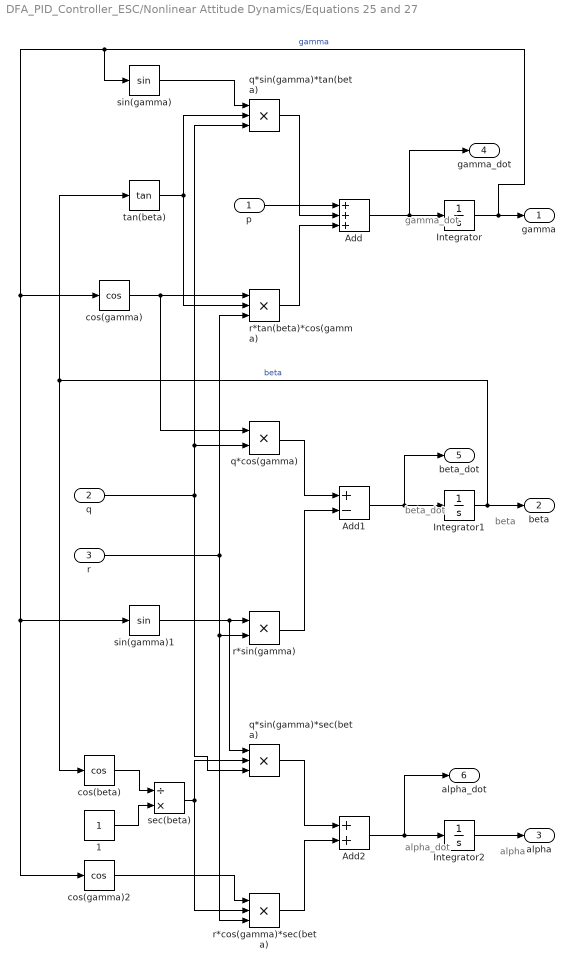
== system DFA_PID_Controller_ESC/Nonlinear Attitude Dynamics/Equations 25 and 27 ==
  note: alpha_dot
  note: alpha
  note: beta_dot
  note: beta
  note: gamma_dot
  p : Inport
  q : Inport  Port=2
  r : Inport  Port=3
  1 : Constant
  Add : Sum  Inputs=+++
  Add1 : Sum  Inputs=+-
  Add2 : Sum
  Integrator : Integrator  InitialCondition=gamma0
  Integrator1 : Integrator  InitialCondition=beta0
  Integrator2 : Integrator  InitialCondition=alpha0
  cos(beta) : Trigonometry  Operator=cos
  cos(gamma) : Trigonometry  Operator=cos
  cos(gamma)2 : Trigonometry  Operator=cos
  q*cos(gamma) : Product  RndMeth=Zero
  q*sin(gamma)*sec(beta) : Product  Inputs=3  RndMeth=Zero
  q*sin(gamma)*tan(beta) : Product  Inputs=3  RndMeth=Zero
  r*cos(gamma)*sec(beta) : Product  Inputs=3  RndMeth=Zero
  r*sin(gamma) : Product  RndMeth=Zero
  r*tan(beta)*cos(gamma) : Product  Inputs=3  RndMeth=Zero
  sec(beta) : Product  Inputs=/*
  sin(gamma) : Trigonometry
  sin(gamma)1 : Trigonometry
  tan(beta) : Trigonometry  Operator=tan
  gamma : Outport
  beta : Outport  Port=2
  alpha : Outport  Port=3
  gamma_dot : Outport  Port=4
  beta_dot : Outport  Port=5
  alpha_dot : Outport  Port=6
  wires:
  cos(beta)/1 -> sec(beta)/1
  sec(beta)/1 -> q*sin(gamma)*sec(beta)/2, r*cos(gamma)*sec(beta)/2
  Add2/1 -> Integrator2/1, alpha_dot/1
  r*cos(gamma)*sec(beta)/1 -> Add2/2
  q*sin(gamma)*sec(beta)/1 -> Add2/1
  cos(gamma)2/1 -> r*cos(gamma)*sec(beta)/1
  Integrator2/1 -> alpha/1
  r*sin(gamma)/1 -> Add1/2
  q*cos(gamma)/1 -> Add1/1
  Add1/1 -> Integrator1/1, beta_dot/1
  q/1 -> q*sin(gamma)*sec(beta)/3, q*cos(gamma)/2, q*sin(gamma)*tan(beta)/3
  r/1 -> r*sin(gamma)/2, r*cos(gamma)*sec(beta)/3, r*tan(beta)*cos(gamma)/3
  sin(gamma)1/1 -> q*sin(gamma)*sec(beta)/1, r*sin(gamma)/1
  Integrator1/1 -> beta/1, cos(beta)/1, tan(beta)/1  "beta"
  Add/1 -> Integrator/1, gamma_dot/1
  q*sin(gamma)*tan(beta)/1 -> Add/2
  r*tan(beta)*cos(gamma)/1 -> Add/3
  p/1 -> Add/1
  tan(beta)/1 -> r*tan(beta)*cos(gamma)/2, q*sin(gamma)*tan(beta)/2
  cos(gamma)/1 -> q*cos(gamma)/1, r*tan(beta)*cos(gamma)/1
  sin(gamma)/1 -> q*sin(gamma)*tan(beta)/1
  Integrator/1 -> cos(gamma)/1, sin(gamma)1/1, cos(gamma)2/1, sin(gamma)/1, gamma/1  "gamma"
  1/1 -> sec(beta)/2

== matlab function DFA_PID_Controller_ESC/IR Sensor/Z Noise ==
  data: u input; y output; IR_mean input; sz input; SENS_NOISE01 input
function y = IRnoise(u,IR_mean,sz, SENS_NOISE01)
r = 0;

if SENS_NOISE01 == 1
r = IR_mean + sz*randn;
end
y = u + r;

== matlab function DFA_PID_Controller_ESC/3D Motion Capture System/X Noise ==
  data: u input; y output; ThreeD_mean input; sx input; SENS_NOISE01 input
function y = ThreeD(u,ThreeD_mean, sx, SENS_NOISE01)

r=0;

if SENS_NOISE01 == 1
    r = ThreeD_mean + sx*randn;
end


y = u + r;

== matlab function DFA_PID_Controller_ESC/IR Sensor/Z_dot Noise ==
  data: u input; y output; IR_mean input; sz input; SENS_NOISE01 input
function y = IRnoise(u,IR_mean,sz, SENS_NOISE01)
r = 0;
if SENS_NOISE01 == 1
r = IR_mean + sz*randn;
end
y = u + r;

== matlab function DFA_PID_Controller_ESC/Nonlinear Attitude Dynamics/Equation 13/angles_1 ==
  data: alpha input; A output; beta input; gamma input
function A  = angles_1(alpha, beta, gamma)
% DFA equations of motion (x-direction)
A = (cos(alpha).*sin(beta).*cos(gamma)) + (sin(alpha).*sin(gamma));
return

== matlab function DFA_PID_Controller_ESC/Nonlinear Attitude Dynamics/Equation 14/angles_2 ==
  data: alpha input; B output; beta input; gamma input
function B  = angles_2(alpha, beta, gamma)
% DFA equations of motion (y-direction)
B = (sin(alpha).*sin(beta).*cos(gamma)) - (cos(alpha).*sin(gamma));
return

== matlab function DFA_PID_Controller_ESC/Nonlinear Attitude Dynamics/Equation 15/angles_3 ==
  data: C output; beta input; gamma input
function C  = angles_3 (beta, gamma)
% DFA equations of motion (z-direction)
C = cos(beta).*cos(gamma);
return

== matlab function DFA_PID_Controller_ESC/3D Motion Capture System/Y_dot Noise ==
  data: u input; y output; ThreeD_mean input; sydot input; SENS_NOISE01 input
function y = ThreeD2(u,ThreeD_mean,sydot,SENS_NOISE01)
%#codegen
r = 0; 
if SENS_NOISE01 == 1
    r = ThreeD_mean + sydot*randn;
end
y = u + r;

== matlab function DFA_PID_Controller_ESC/3D Motion Capture System/X_dot Noise ==
  data: u input; y output; ThreeD_mean input; sxdot input; SENS_NOISE01 input
function y = ThreeD2(u,ThreeD_mean,sxdot,SENS_NOISE01)
%#codegen
r=0;
if SENS_NOISE01==1
    r = ThreeD_mean + sxdot*randn;
end
y = u + r;

== matlab function DFA_PID_Controller_ESC/3D Motion Capture System/Y Noise ==
  data: u input; y output; ThreeD_mean input; sy input; SENS_NOISE01 input
function y = ThreeD(u,ThreeD_mean, sy, SENS_NOISE01)
r=0;
if SENS_NOISE01 == 1
    r = ThreeD_mean + sy*randn;
end
y = u + r;

== matlab function DFA_PID_Controller_ESC/Gyroscope/Gamma Noise ==
  data: u input; y output; Gyromean input; sgamma input; SENS_NOISE01 input
function y = IRnoise(u,Gyromean,sgamma, SENS_NOISE01)
r = 0;
if SENS_NOISE01 == 1
r = Gyromean + sgamma*randn;
end
y = u + r;

== matlab function DFA_PID_Controller_ESC/Accelerometer/Beta_dot Noise ==
  data: u input; y output; Accelmean input; sbetadot input; SENS_NOISE01 input
function y = Accelnoise(u,Accelmean,sbetadot, SENS_NOISE01)
r = 0;
if SENS_NOISE01 == 1
r = Accelmean + sbetadot*randn;
end
y = u + r;

== matlab function DFA_PID_Controller_ESC/Accelerometer/Gamma_dot Noise ==
  data: u input; y output; Accelmean input; sgammadot input; SENS_NOISE01 input
function y = Accelnoise(u,Accelmean,sgammadot, SENS_NOISE01)
r = 0;
if SENS_NOISE01 == 1
r = Accelmean + sgammadot*randn;
end
y = u + r;

== matlab function DFA_PID_Controller_ESC/Accelerometer/Alpha_dot Noise ==
  data: u input; y output; Accelmean input; salphadot input; SENS_NOISE01 input
function y = Accelnoise(u,Accelmean,salphadot, SENS_NOISE01)
r = 0;
if SENS_NOISE01 == 1
r = Accelmean + salphadot*randn;
end
y = u + r;
return

== matlab function DFA_PID_Controller_ESC/Gyroscope/Beta Noise ==
  data: u input; y output; Gyromean input; sbeta input; SENS_NOISE01 input
function y = IRnoise(u,Gyromean,sbeta, SENS_NOISE01)
r = 0;
if SENS_NOISE01 == 1
r = Gyromean + sbeta*randn;
end
y = u + r;

== matlab function DFA_PID_Controller_ESC/Gyroscope/Alpha Noise ==
  data: u input; y output; Gyromean input; salpha input; SENS_NOISE01 input
function y = Gyronoise(u,Gyromean,salpha, SENS_NOISE01)
r = 0;
if SENS_NOISE01 == 1
r = Gyromean + salpha*randn;
end
y = u + r;

== matlab function DFA_PID_Controller_ESC/ESC1 ==
  data: poly_order input; u1 input; ctrl_eff1 output
function ctrl_eff1  = ESC1(poly_order, u1)

ctrl_eff1 = 0;
u1 = u1 + 164;

%Saturate
if(u1 > 255)
    u1 = 255;
end

if(u1 < 0)
    u1 = 0;
end

%Calculate Thrust
if(poly_order == 1)
    ctrl_eff1 = .02317881*u1 - 2.002914;
elseif(poly_order == 2)
    ctrl_eff1 = (-4.6377e-5)*(u1^2) + .03709*u1 - 2.90594;
end

== matlab function DFA_PID_Controller_ESC/MATLAB Function ==
  data: y1 output; y2 output; y3 output; y4 output
function [y1,y2,y3,y4] = fcn()
%#codegen
y1=0;
y2=0;
y3=0;
y4=0;
coder.extrinsic('getjoy'); 
%a=struct('axes',{},'buttons',{},'hats',[]);
[y1,y2,y3,y4]=getjoy();
end

== matlab function DFA_PID_Controller_ESC/ESC2 ==
  data: poly_order input; u2 input; ctrl_eff2 output
function ctrl_eff2 = ESC2(poly_order, u2)

ctrl_eff2 = 0;
u2 = u2 + 164;

%Saturate
if(u2 > 255)
    u2 = 255;
end

if(u2 < 0)
    u2 = 0;
end

%Calculate Thrust
if(poly_order == 1)
    ctrl_eff2 = .02317881*u2 - 2.002914;
elseif(poly_order == 2)
    ctrl_eff2 = (-4.6377e-5)*(u2^2) + .03709*u2 - 2.90594;
end

== matlab function DFA_PID_Controller_ESC/ESC3 ==
  data: poly_order input; u3 input; ctrl_eff3 output
function ctrl_eff3 = ESC3(poly_order, u3)

ctrl_eff3 = 0;
u3 = u3 + 164;

%Saturate
if(u3 > 255)
    u3 = 255;
end

if(u3 < 0)
    u3 = 0;
end

%Calculate Thrust
if(poly_order == 1)
    ctrl_eff3 = .02317881*u3 - 2.002914;
elseif(poly_order == 2)
    ctrl_eff3 = (-4.6377e-5)*(u3^2) + .03709*u3 - 2.90594;
end

== matlab function DFA_PID_Controller_ESC/ESC4 ==
  data: poly_order input; u4 input; ctrl_eff4 output
function ctrl_eff4 = ESC4(poly_order, u4)

ctrl_eff4 = 0;
u4 = u4 + 164;

%Saturate
if(u4 > 255)
    u4 = 255;
end

if(u4 < 0)
    u4 = 0;
end

%Calculate Thrust
if(poly_order == 1)
    ctrl_eff4 = .02317881*u4 - 2.002914;
elseif(poly_order == 2)
    ctrl_eff4 = (-4.6377e-5)*(u4^2) + .03709*u4 - 2.90594;
end

== matlab function DFA_PID_Controller_ESC/MATLAB Function1 ==
  data: u input; y output
function y = TimerFunction(u)
%#codegen

y = 0;

y = u + .01;  %Tstep

if(y >= .21)   %Tpause
    y = 0;
end

== matlab function DFA_PID_Controller_ESC/PID Controller/MATLAB Function ==
  data: beta_d_no_sat input; beta_desired output; gamma_d_no_sat input; gamma_desired output
function [beta_desired, gamma_desired]= AngleSaturate(beta_d_no_sat, gamma_d_no_sat)

beta_desired = beta_d_no_sat;
gamma_desired = gamma_d_no_sat;

if(beta_desired > 1)
    beta_desired = 1;
elseif(beta_desired < -1)
    beta_desired = -1;
end

if(gamma_desired > 1)
    gamma_desired = 1;
elseif(gamma_desired < -1)
    gamma_desired = -1;
end

return
